simulink model "WindowsiCreate"  (R2013a)
settings: Solver=ode3  StartTime=0.0  StopTime=inf  FixedStep=0.01  RelTol=1e-3
undefined symbols (not defined in the file): serial
libraries: instrumentlib x4, vrlib x1, aerolibanimutils x1
settings Model: Creator=Admin  LastModifiedBy=Admin

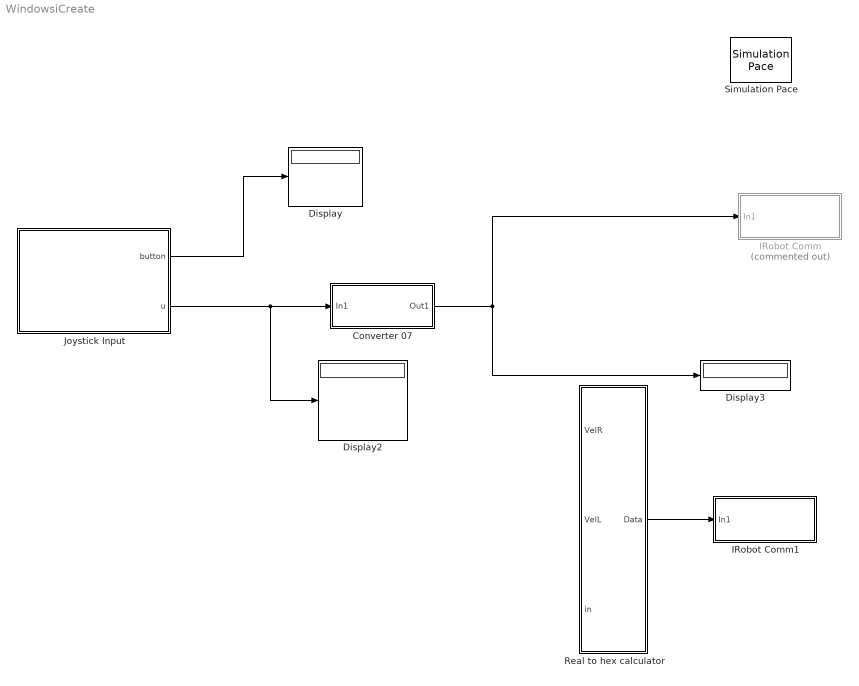
== system WindowsiCreate ==
  Converter 07 : Subsystem
  Display : Display
  Display2 : Display
  Display3 : Display
  IRobot Comm : Subsystem  Commented=on
  IRobot Comm1 : Subsystem
  Joystick Input : Subsystem
  Real to hex calculator : MATLAB Function  TreatAsAtomicUnit=on
  Simulation Pace : aerolibanimutils/Simulation Pace  SimulationPace=1  SleepMode=MATLAB Thread  OutputPaceError=off  SampleTime=-1
      settings: AttributesFormatString=%<SimulationPace> sec/sec
  wires:
  Joystick Input/1(button) -> Display/1
  Converter 07/1(Out1) -> Display3/1, IRobot Comm/1(In1)
  Joystick Input/2(u) -> Display2/1, Converter 07/1(In1)
  Real to hex calculator/1(Data) -> IRobot Comm1/1(In1)

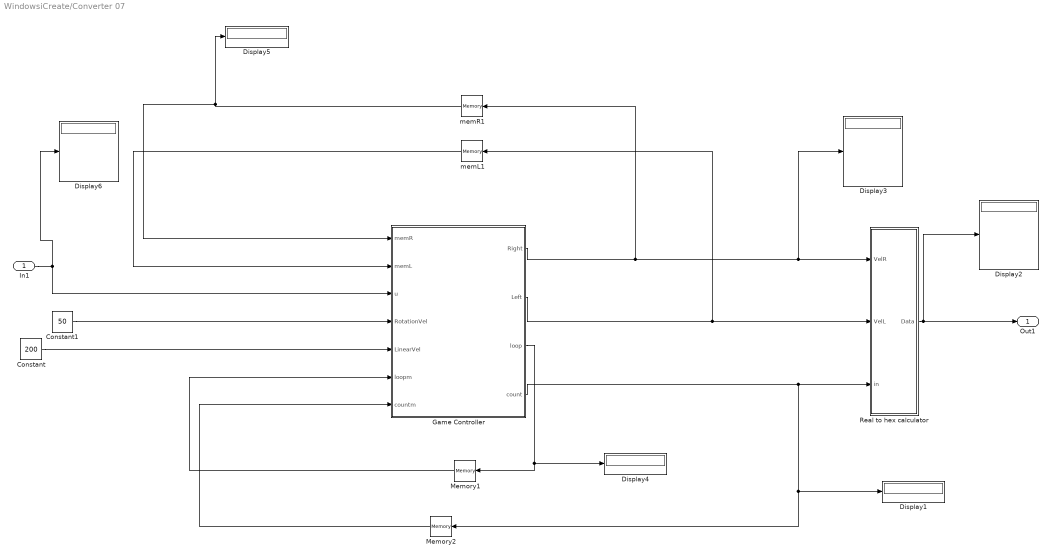
== system WindowsiCreate/Converter 07 ==
  In1 : Inport
  Constant : Constant  Value=200
  Constant1 : Constant  Value=50
  Display{1..6} (6 alike) : Display
  Game Controller : MATLAB Function  TreatAsAtomicUnit=on
  Memory1 : Memory
  Memory2 : Memory
  Real to hex calculator : MATLAB Function  TreatAsAtomicUnit=on
  memL1 : Memory
  memR1 : Memory
  Out1 : Outport
  wires:
  Game Controller/1(Right) -> memR1/1, Display3/1, Real to hex calculator/1(VelR)
  Game Controller/2(Left) -> memL1/1, Real to hex calculator/2(VelL)
  Game Controller/4(count) -> Display1/1, Memory2/1, Real to hex calculator/3(in)
  Real to hex calculator/1(Data) -> Out1/1, Display2/1
  In1/1 -> Display6/1, Game Controller/3(u)
  memR1/1 -> Display5/1, Game Controller/1(memR)
  memL1/1 -> Game Controller/2(memL)
  Constant/1 -> Game Controller/5(LinearVel)
  Constant1/1 -> Game Controller/4(RotationVel)
  Memory2/1 -> Game Controller/7(countm)
  Game Controller/3(loop) -> Display4/1, Memory1/1
  Memory1/1 -> Game Controller/6(loopm)

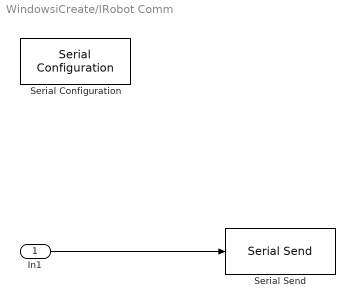
== system WindowsiCreate/IRobot Comm ==
  In1 : Inport
  Serial Configuration : instrumentlib/Serial Configuration  Priority=-200000  ComPortMenu=<Please select a port...>  ComPort=COM4  ObjConstructor=serial('COM4');  BaudRate=57600  DataBits=8  Parity=none  StopBits=1  FlowControl=none  Timeout=10  ByteOrder=LittleEndian
  Serial Send : instrumentlib/Serial Send  ComPortMenu=<Please select a port...>  ComPort=COM4  ObjConstructor=serial('COM4');  Terminator=<none>  EnableBlockingMode=off
  wires:
  In1/1 -> Serial Send/1

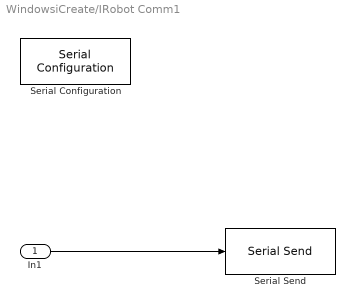
== system WindowsiCreate/IRobot Comm1 ==
  In1 : Inport
  Serial Configuration : instrumentlib/Serial Configuration  Priority=-200000  ComPortMenu=COM3  ComPort=COM3  ObjConstructor=serial('COM3');  BaudRate=57600  DataBits=8  Parity=none  StopBits=1  FlowControl=none  Timeout=10  ByteOrder=LittleEndian
  Serial Send : instrumentlib/Serial Send  ComPortMenu=COM3  ComPort=COM3  ObjConstructor=serial('COM3');  Terminator=<none>  EnableBlockingMode=off
  wires:
  In1/1 -> Serial Send/1

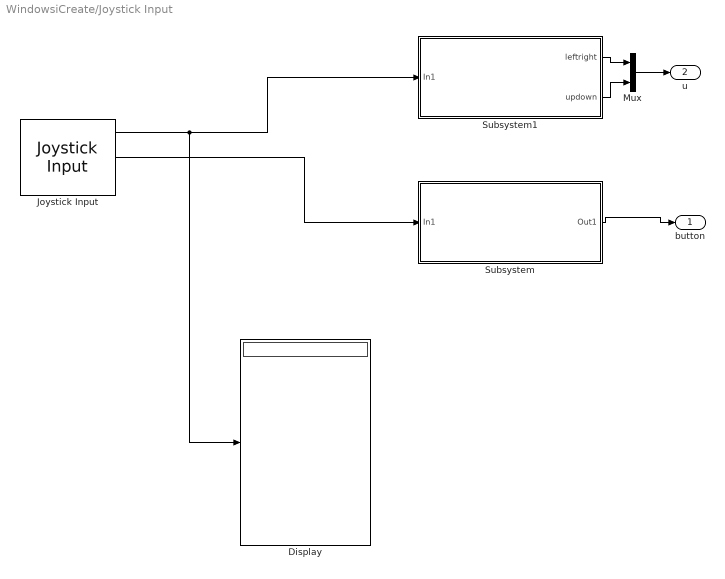
== system WindowsiCreate/Joystick Input ==
  Display : Display
  Joystick Input : vrlib/Joystick Input  joyid=1  adjustports=on  forcefeed=off
  Mux : Mux  Inputs=2
  Subsystem : Subsystem
  Subsystem1 : Subsystem
  button : Outport
  u : Outport  Port=2
  wires:
  Subsystem/1(Out1) -> button/1
  Mux/1 -> u/1
  Subsystem1/1(leftright) -> Mux/1
  Subsystem1/2(updown) -> Mux/2
  Joystick Input/1 -> Subsystem1/1(In1), Display/1
  Joystick Input/2 -> Subsystem/1(In1)

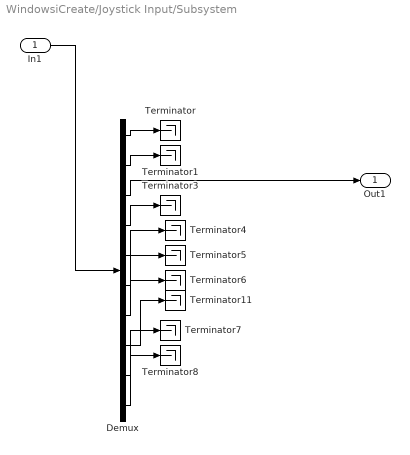
== system WindowsiCreate/Joystick Input/Subsystem ==
  In1 : Inport
  Demux : Demux  Outputs=10
  Terminator{,1,3..8,11} (9 alike) : Terminator
  Out1 : Outport
  wires:
  In1/1 -> Demux/1
  Demux/1 -> Terminator/1
  Demux/2 -> Terminator1/1
  Demux/3 -> Out1/1
  Demux/4 -> Terminator3/1
  Demux/5 -> Terminator4/1
  Demux/9 -> Terminator7/1
  Demux/10 -> Terminator8/1
  Demux/6 -> Terminator5/1
  Demux/7 -> Terminator6/1
  Demux/8 -> Terminator11/1

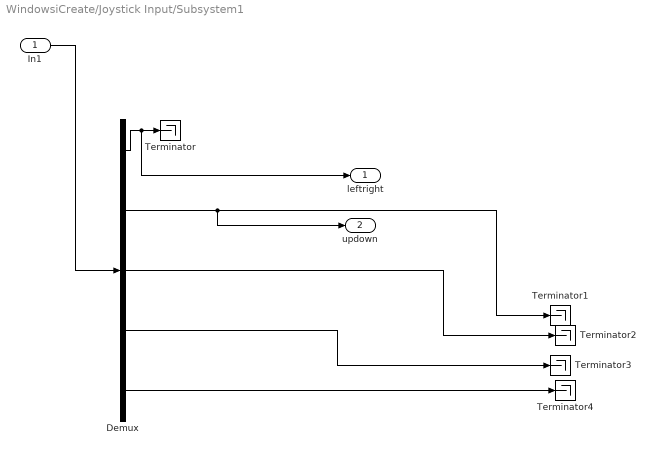
== system WindowsiCreate/Joystick Input/Subsystem1 ==
  In1 : Inport
  Demux : Demux  Outputs=5
  Terminator{,1..4} (5 alike) : Terminator
  leftright : Outport
  updown : Outport  Port=2
  wires:
  Demux/5 -> Terminator4/1
  Demux/4 -> Terminator3/1
  Demux/2 -> updown/1, Terminator1/1
  Demux/1 -> leftright/1, Terminator/1
  In1/1 -> Demux/1
  Demux/3 -> Terminator2/1

== matlab function WindowsiCreate/Converter 07/Game Controller ==
  data: memR input; memL input; u input; RotationVel input; LinearVel input; loopm input; countm input; Right output; Left output; loop output; count output
function [Right,Left,loop,count] = fcn(memR,memL,u,RotationVel,LinearVel,loopm,countm)
% This block supports the Embedded MATLAB subset.
% See the help menu for details. 

%Converts Joystic commands in velocities
if u(1)==1; %turn right
Right=-RotationVel;
Left=RotationVel;
elseif u(1)==-1;%turn left   
Right=RotationVel;
Left=-RotationVel;
else
Right=0;
Left=0;  
end
    
if u(2)==1; %backwards
Right=-LinearVel+Right;
Left=-LinearVel+Left;
elseif u(2)==-1;%forward   
Right=LinearVel+Right;
Left=LinearVel+Left;
else %stop   
Right=Right;
Left=Left;
end 


%Enables a counter to hold inputs and use the serial port in 7 steps

if loopm==0
    
    if Right==memR && Left==memL
        loop=0;
        count=0;
        Right=Right;
        Left=Left;
    else
        loop=1;
        count=1;
        Right=Right;
        Left=Left;
    end
    
else
    if countm==7
        loop=0;
        count=0;
        Right=Right; %refresch Inputs
        Left=Left;
    else
        loop=1;
        count=countm+1;
        Right=memR; %refresch Inputs
        Left=memL;
    end
end

== matlab function WindowsiCreate/Converter 07/Real to hex calculator ==
  data: VelR input; VelL input; Data output; in input
function Data  = fcn(VelR,VelL,in)
% Alessio Grompone january 2014
% Spacecraft Robotics Laboratory, Naval Postgraduate School

%Converts Wheels velocities first to hex then to two decimals as required by iRobot Create

%Right Wheel Conversion
%hiR,lowR,hiL,lowL
DataV=zeros([1,7]);
if VelR>0
    %decimal to numeric hex vector
    A=zeros(4,1);
    B=zeros(4,1);
    d=VelR;
    i=1;
    while d>16
        A(i)=rem(d,16);
        d=floor(d/16);
        i=i+1;
    end
    A(i)=d; %inverted numeric hex vector
    l=size(A);
    n=l(1)+1;
    for z=1:4
        B(z)=A(n-z);
    end
    %numeric hex vector to 2 decimal values
    hiR=B(1)*16+B(2);
    lowR=B(3)*16+B(4);
elseif VelR<0
    uneg=VelR+2^16;
    A=zeros(4,1);
    B=zeros(4,1);
    d=uneg;
    i=1;
    while d>16
        A(i)=rem(d,16);
        d=floor(d/16);
        i=i+1;
    end
    A(i)=d; %inverted numeric hex vector
    l=size(A);
    n=l(1);
    for z=0:n-1
        B(z+1)=A(n-z);
    end
    %numeric hex vector to 2 decimal values
    hiR=B(1)*16+B(2);
    lowR=B(3)*16+B(4);
else
    uneg=VelR+2^16;
    A=zeros(4,1);
    B=zeros(4,1);
    d=uneg;
    i=1;
    hiR=0;
    lowR=0;  
end

if VelL>0
    %decimal to numeric hex vector
    Al=zeros(4,1);
    Bl=zeros(4,1);
    dl=VelL;
    il=1;
    while dl>16
        Al(il)=rem(dl,16);
        dl=floor(dl/16);
        il=il+1;
    end
    Al(il)=dl; %inverted numeric hex vector
    ll=size(Al);
    nl=ll(1)+1;
    for zl=1:4
        Bl(zl)=Al(nl-zl);
    end
    %numeric hex vector to 2 decimal values
    hiL=Bl(1)*16+Bl(2);
    lowL=Bl(3)*16+Bl(4);
elseif VelL<0
    unegl=VelL+2^16;
    Al=zeros(4,1);
    Bl=zeros(4,1);
    dl=unegl;
    il=1;
    while dl>16
        Al(il)=rem(dl,16);
        dl=floor(dl/16);
        il=il+1;
    end
    Al(il)=dl; %inverted numeric hex vector
    ll=size(Al);
    nl=ll(1);
    for zl=0:nl-1
        Bl(zl+1)=Al(nl-zl);
    end
    %numeric hex vector to 2 decimal values
    hiL=Bl(1)*16+Bl(2);
    lowL=Bl(3)*16+Bl(4);
else
    unegl=VelL+2^16;
    Al=zeros(4,1);
    Bl=zeros(4,1);
    dl=unegl;
    il=1;
    hiL=0;
    lowL=0;
end



DataV(1)=128;
DataV(2)=131;
DataV(3)=145;
DataV(4)=hiR;
DataV(5)=lowR;
DataV(6)=hiL;
DataV(7)=lowL;

if in>0
Data=DataV(in);
else
Data=0;
end

== matlab function WindowsiCreate/Real to hex calculator ==
  data: VelR input; VelL input; Data output; in input
function Data  = fcn(VelR,VelL,in)
% Alessio Grompone january 2014
% Spacecraft Robotics Laboratory, Naval Postgraduate School

%Converts Wheels velocities first to hex then to two decimals as required by iRobot Create

%Right Wheel Conversion
%hiR,lowR,hiL,lowL
DataV=zeros([1,7]);
if VelR>0
    %decimal to numeric hex vector
    A=zeros(4,1);
    B=zeros(4,1);
    d=VelR;
    i=1;
    while d>16
        A(i)=rem(d,16);
        d=floor(d/16);
        i=i+1;
    end
    A(i)=d; %inverted numeric hex vector
    l=size(A);
    n=l(1)+1;
    for z=1:4
        B(z)=A(n-z);
    end
    %numeric hex vector to 2 decimal values
    hiR=B(1)*16+B(2);
    lowR=B(3)*16+B(4);
elseif VelR<0
    uneg=VelR+2^16;
    A=zeros(4,1);
    B=zeros(4,1);
    d=uneg;
    i=1;
    while d>16
        A(i)=rem(d,16);
        d=floor(d/16);
        i=i+1;
    end
    A(i)=d; %inverted numeric hex vector
    l=size(A);
    n=l(1);
    for z=0:n-1
        B(z+1)=A(n-z);
    end
    %numeric hex vector to 2 decimal values
    hiR=B(1)*16+B(2);
    lowR=B(3)*16+B(4);
else
    uneg=VelR+2^16;
    A=zeros(4,1);
    B=zeros(4,1);
    d=uneg;
    i=1;
    hiR=0;
    lowR=0;  
end

if VelL>0
    %decimal to numeric hex vector
    Al=zeros(4,1);
    Bl=zeros(4,1);
    dl=VelL;
    il=1;
    while dl>16
        Al(il)=rem(dl,16);
        dl=floor(dl/16);
        il=il+1;
    end
    Al(il)=dl; %inverted numeric hex vector
    ll=size(Al);
    nl=ll(1)+1;
    for zl=1:4
        Bl(zl)=Al(nl-zl);
    end
    %numeric hex vector to 2 decimal values
    hiL=Bl(1)*16+Bl(2);
    lowL=Bl(3)*16+Bl(4);
elseif VelL<0
    unegl=VelL+2^16;
    Al=zeros(4,1);
    Bl=zeros(4,1);
    dl=unegl;
    il=1;
    while dl>16
        Al(il)=rem(dl,16);
        dl=floor(dl/16);
        il=il+1;
    end
    Al(il)=dl; %inverted numeric hex vector
    ll=size(Al);
    nl=ll(1);
    for zl=0:nl-1
        Bl(zl+1)=Al(nl-zl);
    end
    %numeric hex vector to 2 decimal values
    hiL=Bl(1)*16+Bl(2);
    lowL=Bl(3)*16+Bl(4);
else
    unegl=VelL+2^16;
    Al=zeros(4,1);
    Bl=zeros(4,1);
    dl=unegl;
    il=1;
    hiL=0;
    lowL=0;
end



DataV(1)=128;
DataV(2)=131;
DataV(3)=145;
DataV(4)=hiR;
DataV(5)=lowR;
DataV(6)=hiL;
DataV(7)=lowL;

if in>0
Data=DataV(in);
else
Data=0;
end
